simulink model "CARNOTews_M10C5_V1"  (Simulink 7.6)
settings: Solver=ode23tb  StartTime=t0  StopTime=t1
InitFcn:
  | tic;
  | parameter_CARNOTews;
StopFcn:
  | save(myfile,'simout');
  | save(myfile1,'simout1');
  | disp(['t_sim = ' num2str(toc/60) ' min'])
undefined symbols (not defined in the file or in its folder): Ad, Ad0, Ar, Au, Au0, Bd, Bd0, Bohrdurchmesser, Br, Bu, Bu0, c1, c33, c4, Cd, Cdl, Cr, Cu, Dd, DimAxi, DimRad, Dl, Dr, Du, fluid, gfunction, Gitterfaktor, Jahresmitteltemp, L1, lambdaErde, Massenstrom, mdot, mix, np, p0, Rechenradius, sample_time, Sondelaenge, Sondendurchmesser, T_null, t_start, Tdown_0, Tearth_anf, teta_in, TGrad, Ts_Trichter, Tup_0
libraries: carnot x2, simulink x1
settings Model: Creator=c8461075  LastModifiedBy=Fabian Ochs  SimulationMode=accelerator
settings OptimizationCC: InlineParams=on  SimCompilerOptimization=On
settings DebuggingCC: FcnCallInpInsideContextMsg=Enable All  UniqueDataStoreMsg=error

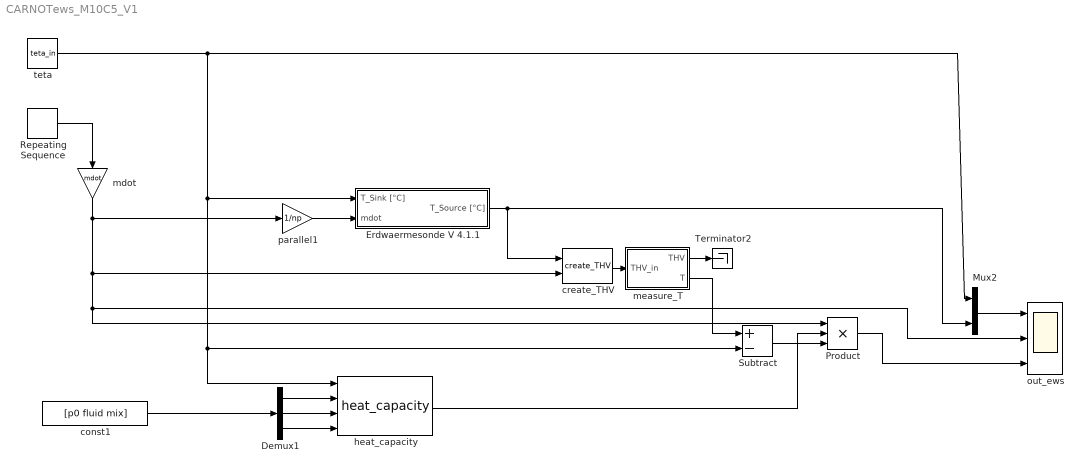
== system CARNOTews_M10C5_V1 ==
  Demux1 : Demux  Outputs=3
  Erdwaermesonde V 4.1.1 : Subsystem  mask{DimAxi=DimAxi, DimRad=DimRad, Jahresmitteltemp=Jahresmitteltemp, TGrad=TGrad, Massenstrom=Massenstrom, Sondendurchmesser=Sondendurchmesser, Bohrdurchmesser=Bohrdurchmesser, Sondelaenge=Sondelaenge, Rechenradius=Rechenradius, Gitterfaktor=Gitterfaktor}
      mask prompts: DimAxi "Knoten in axialer Richtung:"; DimRad "Knoten in radialer Richtung:"; Jahresmitteltemp "Jahresmitteltemperatur (K):"; TGrad "Temperaturgradient (K/m):"; Massenstrom "Massenstrom Sole (Kg/s):"; Sondendurchmesser "Sondendurchmesser (m):"; Bohrdurchmesser "Bohrdurchmesser (m):"; Sondelaenge "Sondenlänge (m):"; Rechenradius "Rechenradius (m):"
      mask help: Erdwärmesonde
      mask Help:
      | Anfangstemperatur T_PA: Verwendet die stationäre Temperaturverteilung der Erde und der Sole als Anfangstemperaturen im ganzen Gitter (Simulation fängt während der Heizsaison an).
      | Falls T_PA=-1 sind die Temperaturen der Erde in radialer Richtung konstant (die Simulation fängt am Anfang der Heizsaison an).
  Mux2 : Mux  Inputs=2
  Product : Product  Inputs=3  RndMeth=Zero
  Repeating Sequence : simulink/Sources/Repeating Sequence  SystemSampleTime=-1  rep_seq_t=[0 12 12 24]*3600  rep_seq_y=[1 1 0 0]
  Subtract : Sum  Inputs=+-
  Terminator2 : Terminator
  const1 : Constant  Value=[p0 fluid mix]
  create_THV : carnot/misc/create_THV  SystemSampleTime=-1  p=p0  fluid=water_glycol_mix  mix=mix  dia=0.02
  heat_capacity : carnot/materials/heat_capacity  SystemSampleTime=-1
  mdot : Gain  Gain=mdot
  measure_T : Subsystem  AncestorBlock=carnot/control/measure_T  mask(temperature measurement sensor){tc=10, t0=20}
      mask prompts: tc "time constant of sensor [s]"; t0 "initial temperature [degree centigrade]"
      mask help: Measurement sensor for temperatures with first-oder hold. Temperature is in degree centigrade.
      mask init:
      | tc = 1/max(tc, 0.001);
      mask Help: eval('man (''measure_T'')')
      mask Display: plot(-18,0,30,20,[0 20],[0 0],[10 10 8 8 12 12 10],[0 8 8 17 17 8 8],[10 10 9 9 11 11 10 9],[15 10 10 9 9 10 9 10])
  out_ews : Scope  NumInputPorts=3
      settings: TickLabels=on  YMin=1~0~0  YMax=11~0.5~37500  SaveName=simout  SampleInput=on  SampleTime=sample_time
  parallel1 : Gain  Gain=1/np
  teta : Constant  Value=teta_in
  wires:
  Mux2/1 -> out_ews/1
  Subtract/1 -> Product/3
  parallel1/1 -> Erdwaermesonde V 4.1.1/2(mdot)
  Erdwaermesonde V 4.1.1/1(T_Source [°C]) -> create_THV/1, Mux2/2
  create_THV/1 -> measure_T/1(THV_in)
  measure_T/2(T) -> Subtract/1
  measure_T/1(THV) -> Terminator2/1
  Demux1/1 -> heat_capacity/2
  Demux1/2 -> heat_capacity/3
  Demux1/3 -> heat_capacity/4
  teta/1 -> Erdwaermesonde V 4.1.1/1(T_Sink [°C]), heat_capacity/1, Subtract/2, Mux2/1
  const1/1 -> Demux1/1
  mdot/1 -> parallel1/1, create_THV/2, Product/1, out_ews/2
  heat_capacity/1 -> Product/2
  Product/1 -> out_ews/3
  Repeating Sequence/1 -> mdot/1

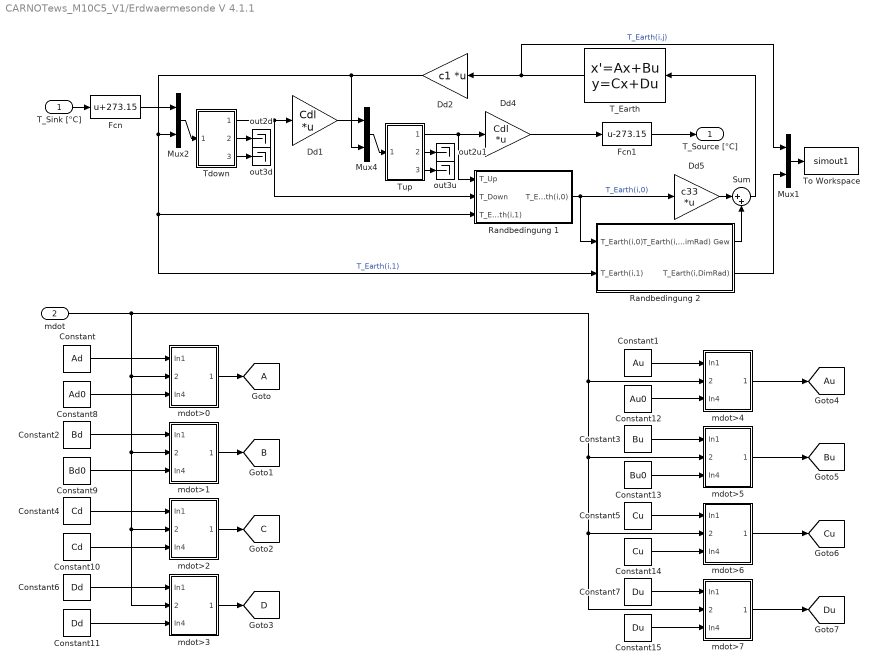
== system CARNOTews_M10C5_V1/Erdwaermesonde V 4.1.1 ==
  T_Sink [°C] : Inport
  mdot : Inport  Port=2
  Constant : Constant  Value=Ad
  Constant1 : Constant  Value=Au
  Constant10 : Constant  Value=Cd
  Constant11 : Constant  Value=Dd
  Constant12 : Constant  Value=Au0
  Constant13 : Constant  Value=Bu0
  Constant14 : Constant  Value=Cu
  Constant15 : Constant  Value=Du
  Constant2 : Constant  Value=Bd
  Constant3 : Constant  Value=Bu
  Constant4 : Constant  Value=Cd
  Constant5 : Constant  Value=Cu
  Constant6 : Constant  Value=Dd
  Constant7 : Constant  Value=Du
  Constant8 : Constant  Value=Ad0
  Constant9 : Constant  Value=Bd0
  Dd1 : Gain  Gain=Cdl  Multiplication=Matrix(K*u)  SaturateOnIntegerOverflow=on  OutDataTypeStr=Inherit: Same as input  ParamDataTypeStr=Inherit: Same as input
  Dd2 : Gain  Gain=c1  Multiplication=Matrix(K*u)  SaturateOnIntegerOverflow=on  OutDataTypeStr=Inherit: Same as input  ParamDataTypeStr=Inherit: Same as input
  Dd4 : Gain  Gain=Cdl  Multiplication=Matrix(K*u)  SaturateOnIntegerOverflow=on  OutDataTypeStr=Inherit: Same as input  ParamDataTypeStr=Inherit: Same as input
  Dd5 : Gain  Gain=c33  Multiplication=Matrix(K*u)  SaturateOnIntegerOverflow=on  OutDataTypeStr=Inherit: Same as input  ParamDataTypeStr=Inherit: Same as input
  Fcn : Fcn  Expr=u+273.15
  Fcn1 : Fcn  Expr=u-273.15
  Mux1 : Mux  Inputs=2
  Mux2 : Mux  Inputs=2
  Mux4 : Mux  Inputs=2
  Randbedingung 1 : Subsystem
  Randbedingung 2 : Subsystem
  Sum : Sum  Inputs=|++  SaturateOnIntegerOverflow=on  InputSameDT=on  OutDataTypeStr=Inherit: Same as first input
  T_Earth : StateSpace  A=Ar  B=Br  C=Cr  D=Dr  X0=Tearth_anf(:)
  Tdown : Subsystem
  To Workspace : ToWorkspace  VariableName=simout1  SampleTime=sample_time  SaveFormat=Structure With Time
  Tup : Subsystem
  mdot>0 : Subsystem
  mdot>1 : Subsystem
  mdot>2 : Subsystem
  mdot>3 : Subsystem
  mdot>4 : Subsystem
  mdot>5 : Subsystem
  mdot>6 : Subsystem
  mdot>7 : Subsystem
  out2d : Terminator
  out2u1 : Terminator
  out3d : Terminator
  out3u : Terminator
  T_Source [°C] : Outport
  tag scope: A=global, Au=global, B=global, Bu=global, C=global, Cu=global, D=global, Du=global
  wires:
  Fcn/1 -> Mux2/1
  Fcn1/1 -> T_Source [°C]/1
  Randbedingung 2/2(T_Earth(i,DimRad)) -> Mux1/2
  Dd2/1 -> Mux2/2, Randbedingung 1/3(T_Earth(i,1)), Randbedingung 2/2(T_Earth(i,1)), Mux4/2  "T_Earth(i,1)"
  Randbedingung 1/1(T_Earth(i,0)) -> Randbedingung 2/1(T_Earth(i,0)), Dd5/1  "T_Earth(i,0)"
  T_Sink [°C]/1 -> Fcn/1
  Sum/1 -> T_Earth/1
  Randbedingung 2/1(T_Earth(i,DimRad) Gew) -> Sum/2
  Dd5/1 -> Sum/1
  Dd4/1 -> Fcn1/1
  Tup/1(Out1) -> Dd4/1, Randbedingung 1/1(T_Up)
  T_Earth/1 -> Dd2/1, Mux1/1  "T_Earth(i,j)"
  Dd1/1 -> Mux4/1
  Mux4/1 -> Tup/1(In1)
  Mux2/1 -> Tdown/1(In1)
  Tdown/1(Out1) -> Dd1/1, Randbedingung 1/2(T_Down)
  Tdown/3(Out3) -> out3d/1
  Tup/3(Out3) -> out3u/1
  Tdown/2(Out2) -> out2d/1
  Tup/2(Out2) -> out2u1/1
  mdot>0/1(Out1) -> [A]
  Constant8/1 -> mdot>0/3(In4)
  mdot>1/1(Out1) -> [B]
  Constant/1 -> mdot>0/1(In1)
  Constant2/1 -> mdot>1/1(In1)
  Constant9/1 -> mdot>1/3(In4)
  mdot>2/1(Out1) -> [C]
  Constant4/1 -> mdot>2/1(In1)
  mdot>3/1(Out1) -> [D]
  Constant10/1 -> mdot>2/3(In4)
  Constant11/1 -> mdot>3/3(In4)
  Constant6/1 -> mdot>3/1(In1)
  Constant1/1 -> mdot>4/1(In1)
  Constant3/1 -> mdot>5/1(In1)
  Constant5/1 -> mdot>6/1(In1)
  Constant7/1 -> mdot>7/1(In1)
  mdot>7/1(Out1) -> [Du]
  mdot>6/1(Out1) -> [Cu]
  mdot>5/1(Out1) -> [Bu]
  mdot>4/1(Out1) -> [Au]
  Constant15/1 -> mdot>7/3(In4)
  Constant14/1 -> mdot>6/3(In4)
  Constant13/1 -> mdot>5/3(In4)
  Constant12/1 -> mdot>4/3(In4)
  mdot/1 -> mdot>0/2(mdot), mdot>1/2(mdot), mdot>2/2(mdot), mdot>3/2(mdot), mdot>4/2(mdot), mdot>5/2(mdot), mdot>6/2(mdot), mdot>7/2(mdot)
  Mux1/1 -> To Workspace/1

== system CARNOTews_M10C5_V1/measure_T ==
  THV_in : Inport
  heat capacity : StateSpace  A=-tc  B=tc  D=0  X0=t0
  select temperature : Selector  InputPortWidth=20  IndexOptions=Index vector (dialog)  Indices=[2]  OutputSizes=1
  THV : Outport  InitialOutput=0
  T : Outport  Port=2  InitialOutput=0
  wires:
  THV_in/1 -> select temperature/1, THV/1
  select temperature/1 -> heat capacity/1
  heat capacity/1 -> T/1

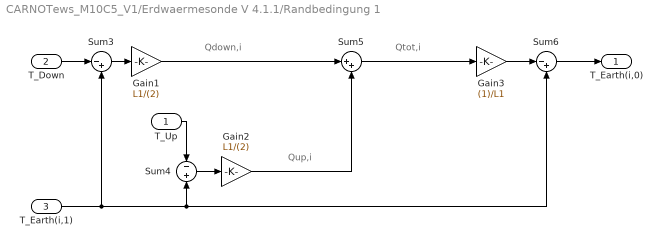
== system CARNOTews_M10C5_V1/Erdwaermesonde V 4.1.1/Randbedingung 1 ==
  note: Qtot,i
  note: Qup,i
  note: Qdown,i
  T_Up : Inport
  T_Down : Inport  Port=2
  T_Earth(i,1) : Inport  Port=3
  Gain1 : Gain  Gain=L1/(2)  SaturateOnIntegerOverflow=on  OutDataTypeStr=Inherit: Same as input  ParamDataTypeStr=Inherit: Same as input
  Gain2 : Gain  Gain=L1/(2)  SaturateOnIntegerOverflow=on  OutDataTypeStr=Inherit: Same as input  ParamDataTypeStr=Inherit: Same as input
  Gain3 : Gain  Gain=(1)/L1  SaturateOnIntegerOverflow=on  OutDataTypeStr=Inherit: Same as input  ParamDataTypeStr=Inherit: Same as input
  Sum3 : Sum  Inputs=|-+  SaturateOnIntegerOverflow=on  InputSameDT=on  OutDataTypeStr=Inherit: Same as first input
  Sum4 : Sum  Inputs=-+  SaturateOnIntegerOverflow=on  InputSameDT=on  OutDataTypeStr=Inherit: Same as first input
  Sum5 : Sum  Inputs=|++  SaturateOnIntegerOverflow=on  InputSameDT=on  OutDataTypeStr=Inherit: Same as first input
  Sum6 : Sum  Inputs=|-+  SaturateOnIntegerOverflow=on  InputSameDT=on  OutDataTypeStr=Inherit: Same as first input
  T_Earth(i,0) : Outport
  wires:
  Sum6/1 -> T_Earth(i,0)/1
  T_Earth(i,1)/1 -> Sum6/2, Sum4/2, Sum3/2
  T_Up/1 -> Sum4/1
  T_Down/1 -> Sum3/1
  Gain3/1 -> Sum6/1
  Sum5/1 -> Gain3/1
  Gain2/1 -> Sum5/2
  Gain1/1 -> Sum5/1
  Sum4/1 -> Gain2/1
  Sum3/1 -> Gain1/1

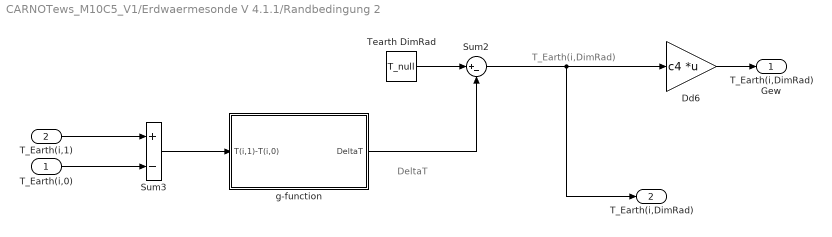
== system CARNOTews_M10C5_V1/Erdwaermesonde V 4.1.1/Randbedingung 2 ==
  note: DeltaT
  note: T_Earth(i,DimRad)
  T_Earth(i,0) : Inport
  T_Earth(i,1) : Inport  Port=2
  Dd6 : Gain  Gain=c4  Multiplication=Matrix(K*u)  SaturateOnIntegerOverflow=on  OutDataTypeStr=Inherit: Same as input  ParamDataTypeStr=Inherit: Same as input
  Sum2 : Sum  Inputs=|+-  SaturateOnIntegerOverflow=on  InputSameDT=on  OutDataTypeStr=Inherit: Same as first input
  Sum3 : Sum  Inputs=+-  SaturateOnIntegerOverflow=on  InputSameDT=on  OutDataTypeStr=Inherit: Same as first input
  Tearth DimRad : Constant  Value=T_null  VectorParams1D=off
  g-function : Subsystem
  T_Earth(i,DimRad) Gew : Outport
  T_Earth(i,DimRad) : Outport  Port=2
  wires:
  g-function/1(DeltaT) -> Sum2/2
  Sum3/1 -> g-function/1(T(i,1)-T(i,0))
  Dd6/1 -> T_Earth(i,DimRad) Gew/1
  T_Earth(i,0)/1 -> Sum3/2
  T_Earth(i,1)/1 -> Sum3/1
  Tearth DimRad/1 -> Sum2/1
  Sum2/1 -> T_Earth(i,DimRad)/1, Dd6/1

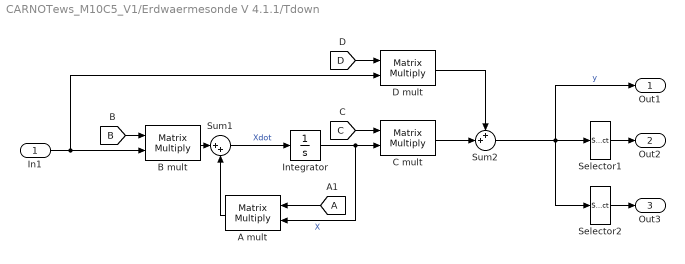
== system CARNOTews_M10C5_V1/Erdwaermesonde V 4.1.1/Tdown ==
  In1 : Inport
  A mult : Product  Multiplication=Matrix(*)  RndMeth=Zero
  B mult : Product  Multiplication=Matrix(*)  RndMeth=Zero
  C mult : Product  Multiplication=Matrix(*)  RndMeth=Zero
  D mult : Product  Multiplication=Matrix(*)  RndMeth=Zero
  Integrator : Integrator  InitialCondition=Tdown_0
  Selector1 : Selector  InputPortWidth=DimAxi/2  IndexOptions=Index vector (dialog)  Indices=1  OutputSizes=1
  Selector2 : Selector  InputPortWidth=DimAxi/2  IndexOptions=Index vector (dialog)  Indices=2  OutputSizes=1
  Sum1 : Sum  Inputs=|++
  Sum2 : Sum  Inputs=++|
  Out1 : Outport
  Out2 : Outport  Port=2
  Out3 : Outport  Port=3
  wires:
  Sum2/1 -> Selector2/1, Selector1/1, Out1/1  "y"
  In1/1 -> B mult/2, D mult/2
  D mult/1 -> Sum2/1
  C mult/1 -> Sum2/2
  B mult/1 -> Sum1/1
  Sum1/1 -> Integrator/1  "Xdot"
  Integrator/1 -> A mult/2, C mult/2  "X"
  A mult/1 -> Sum1/2
  [B] -> B mult/1
  [A] -> A mult/1
  [C] -> C mult/1
  [D] -> D mult/1
  Selector1/1 -> Out2/1
  Selector2/1 -> Out3/1

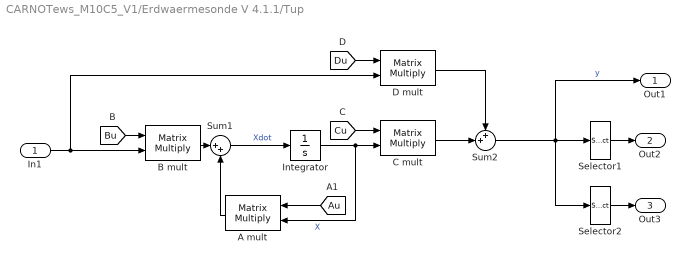
== system CARNOTews_M10C5_V1/Erdwaermesonde V 4.1.1/Tup ==
  In1 : Inport
  A mult : Product  Multiplication=Matrix(*)  RndMeth=Zero
  B mult : Product  Multiplication=Matrix(*)  RndMeth=Zero
  C mult : Product  Multiplication=Matrix(*)  RndMeth=Zero
  D mult : Product  Multiplication=Matrix(*)  RndMeth=Zero
  Integrator : Integrator  InitialCondition=Tup_0
  Selector1 : Selector  InputPortWidth=DimAxi/2  IndexOptions=Index vector (dialog)  Indices=1  OutputSizes=1
  Selector2 : Selector  InputPortWidth=DimAxi/2  IndexOptions=Index vector (dialog)  Indices=2  OutputSizes=1
  Sum1 : Sum  Inputs=|++
  Sum2 : Sum  Inputs=++|
  Out1 : Outport
  Out2 : Outport  Port=2
  Out3 : Outport  Port=3
  wires:
  Sum2/1 -> Selector2/1, Selector1/1, Out1/1  "y"
  In1/1 -> B mult/2, D mult/2
  D mult/1 -> Sum2/1
  C mult/1 -> Sum2/2
  B mult/1 -> Sum1/1
  Sum1/1 -> Integrator/1  "Xdot"
  Integrator/1 -> A mult/2, C mult/2  "X"
  A mult/1 -> Sum1/2
  [Bu] -> B mult/1
  [Au] -> A mult/1
  [Cu] -> C mult/1
  [Du] -> D mult/1
  Selector1/1 -> Out2/1
  Selector2/1 -> Out3/1

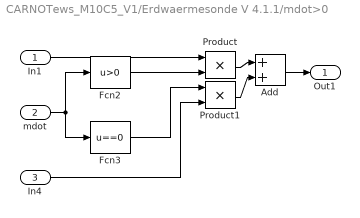
== system CARNOTews_M10C5_V1/Erdwaermesonde V 4.1.1/mdot>0 ==
  In1 : Inport
  mdot : Inport  Port=2
  In4 : Inport  Port=3
  Add : Sum
  Fcn2 : Fcn  Expr=u>0
  Fcn3 : Fcn  Expr=u==0
  Product : Product  RndMeth=Zero
  Product1 : Product  RndMeth=Zero
  Out1 : Outport
  wires:
  Product/1 -> Add/1
  Product1/1 -> Add/2
  In1/1 -> Product/1
  Add/1 -> Out1/1
  In4/1 -> Product1/2
  mdot/1 -> Fcn2/1, Fcn3/1
  Fcn2/1 -> Product/2
  Fcn3/1 -> Product1/1

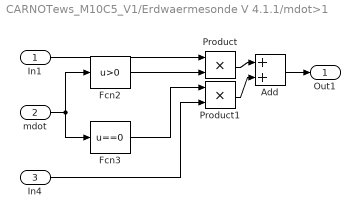
== system CARNOTews_M10C5_V1/Erdwaermesonde V 4.1.1/mdot>1 ==
  In1 : Inport
  mdot : Inport  Port=2
  In4 : Inport  Port=3
  Add : Sum
  Fcn2 : Fcn  Expr=u>0
  Fcn3 : Fcn  Expr=u==0
  Product : Product  RndMeth=Zero
  Product1 : Product  RndMeth=Zero
  Out1 : Outport
  wires:
  Product/1 -> Add/1
  Product1/1 -> Add/2
  In1/1 -> Product/1
  Add/1 -> Out1/1
  In4/1 -> Product1/2
  mdot/1 -> Fcn2/1, Fcn3/1
  Fcn2/1 -> Product/2
  Fcn3/1 -> Product1/1

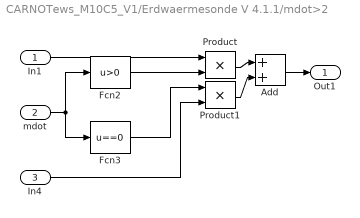
== system CARNOTews_M10C5_V1/Erdwaermesonde V 4.1.1/mdot>2 ==
  In1 : Inport
  mdot : Inport  Port=2
  In4 : Inport  Port=3
  Add : Sum
  Fcn2 : Fcn  Expr=u>0
  Fcn3 : Fcn  Expr=u==0
  Product : Product  RndMeth=Zero
  Product1 : Product  RndMeth=Zero
  Out1 : Outport
  wires:
  Product/1 -> Add/1
  Product1/1 -> Add/2
  In1/1 -> Product/1
  Add/1 -> Out1/1
  In4/1 -> Product1/2
  mdot/1 -> Fcn2/1, Fcn3/1
  Fcn2/1 -> Product/2
  Fcn3/1 -> Product1/1

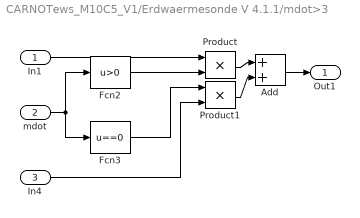
== system CARNOTews_M10C5_V1/Erdwaermesonde V 4.1.1/mdot>3 ==
  In1 : Inport
  mdot : Inport  Port=2
  In4 : Inport  Port=3
  Add : Sum
  Fcn2 : Fcn  Expr=u>0
  Fcn3 : Fcn  Expr=u==0
  Product : Product  RndMeth=Zero
  Product1 : Product  RndMeth=Zero
  Out1 : Outport
  wires:
  Product/1 -> Add/1
  Product1/1 -> Add/2
  In1/1 -> Product/1
  Add/1 -> Out1/1
  In4/1 -> Product1/2
  mdot/1 -> Fcn2/1, Fcn3/1
  Fcn2/1 -> Product/2
  Fcn3/1 -> Product1/1

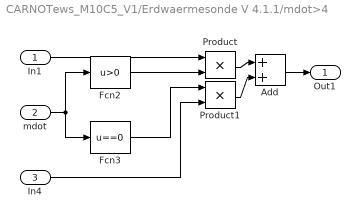
== system CARNOTews_M10C5_V1/Erdwaermesonde V 4.1.1/mdot>4 ==
  In1 : Inport
  mdot : Inport  Port=2
  In4 : Inport  Port=3
  Add : Sum
  Fcn2 : Fcn  Expr=u>0
  Fcn3 : Fcn  Expr=u==0
  Product : Product  RndMeth=Zero
  Product1 : Product  RndMeth=Zero
  Out1 : Outport
  wires:
  Product/1 -> Add/1
  Product1/1 -> Add/2
  In1/1 -> Product/1
  Add/1 -> Out1/1
  In4/1 -> Product1/2
  mdot/1 -> Fcn2/1, Fcn3/1
  Fcn2/1 -> Product/2
  Fcn3/1 -> Product1/1

== system CARNOTews_M10C5_V1/Erdwaermesonde V 4.1.1/mdot>5 ==
  In1 : Inport
  mdot : Inport  Port=2
  In4 : Inport  Port=3
  Add : Sum
  Fcn2 : Fcn  Expr=u>0
  Fcn3 : Fcn  Expr=u==0
  Product : Product  RndMeth=Zero
  Product1 : Product  RndMeth=Zero
  Out1 : Outport
  wires:
  Product/1 -> Add/1
  Product1/1 -> Add/2
  In1/1 -> Product/1
  Add/1 -> Out1/1
  In4/1 -> Product1/2
  mdot/1 -> Fcn2/1, Fcn3/1
  Fcn2/1 -> Product/2
  Fcn3/1 -> Product1/1

== system CARNOTews_M10C5_V1/Erdwaermesonde V 4.1.1/mdot>6 ==
  In1 : Inport
  mdot : Inport  Port=2
  In4 : Inport  Port=3
  Add : Sum
  Fcn2 : Fcn  Expr=u>0
  Fcn3 : Fcn  Expr=u==0
  Product : Product  RndMeth=Zero
  Product1 : Product  RndMeth=Zero
  Out1 : Outport
  wires:
  Product/1 -> Add/1
  Product1/1 -> Add/2
  In1/1 -> Product/1
  Add/1 -> Out1/1
  In4/1 -> Product1/2
  mdot/1 -> Fcn2/1, Fcn3/1
  Fcn2/1 -> Product/2
  Fcn3/1 -> Product1/1

== system CARNOTews_M10C5_V1/Erdwaermesonde V 4.1.1/mdot>7 ==
  In1 : Inport
  mdot : Inport  Port=2
  In4 : Inport  Port=3
  Add : Sum
  Fcn2 : Fcn  Expr=u>0
  Fcn3 : Fcn  Expr=u==0
  Product : Product  RndMeth=Zero
  Product1 : Product  RndMeth=Zero
  Out1 : Outport
  wires:
  Product/1 -> Add/1
  Product1/1 -> Add/2
  In1/1 -> Product/1
  Add/1 -> Out1/1
  In4/1 -> Product1/2
  mdot/1 -> Fcn2/1, Fcn3/1
  Fcn2/1 -> Product/2
  Fcn3/1 -> Product1/1

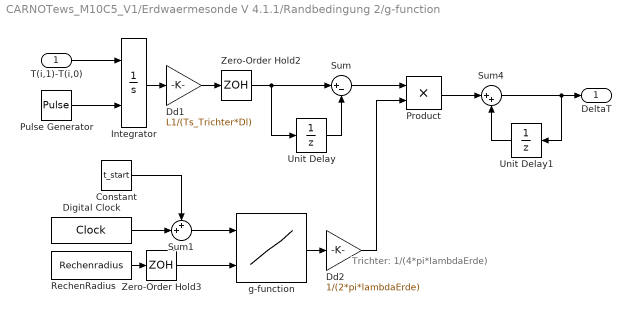
== system CARNOTews_M10C5_V1/Erdwaermesonde V 4.1.1/Randbedingung 2/g-function ==
  note: Trichter: 1/(4*pi*lambdaErde)
  T(i,1)-T(i,0) : Inport
  Constant : Constant  Value=t_start
  Dd1 : Gain  Gain=L1/(Ts_Trichter*Dl)  SaturateOnIntegerOverflow=on  OutDataTypeStr=Inherit: Same as input  ParamDataTypeStr=Inherit: Same as input
  Dd2 : Gain  Gain=1/(2*pi*lambdaErde)  SaturateOnIntegerOverflow=on  OutDataTypeStr=Inherit: Same as input  ParamDataTypeStr=Inherit: Same as input
  Digital Clock : DigitalClock
  Integrator : Integrator  ExternalReset=rising
  Product : Product  SaturateOnIntegerOverflow=on  RndMeth=Zero  InputSameDT=on  OutDataTypeStr=Inherit: Same as first input
  Pulse Generator : DiscretePulseGenerator  PulseType=Time based  Period=Ts_Trichter  PulseWidth=50  PhaseDelay=300
  RechenRadius : Constant  Value=Rechenradius  VectorParams1D=off
  Sum : Sum  Inputs=|+-  SaturateOnIntegerOverflow=on  InputSameDT=on  OutDataTypeStr=Inherit: Same as first input
  Sum1 : Sum  Inputs=++|  SaturateOnIntegerOverflow=on  InputSameDT=on  OutDataTypeStr=Inherit: Same as first input
  Sum4 : Sum  Inputs=|++  SaturateOnIntegerOverflow=on  InputSameDT=on  OutDataTypeStr=Inherit: Same as first input
  Unit Delay : UnitDelay
  Unit Delay1 : UnitDelay
  Zero-Order Hold2 : ZeroOrderHold
  Zero-Order Hold3 : ZeroOrderHold
  g-function : Lookup2D  RowIndex=t_Trichter  ColumnIndex=r_Trichter  Table=gfunction  SaturateOnIntegerOverflow=on  InputSameDT=on
  DeltaT : Outport
  wires:
  T(i,1)-T(i,0)/1 -> Integrator/1
  Zero-Order Hold2/1 -> Sum/1, Unit Delay/1
  Zero-Order Hold3/1 -> g-function/2
  Sum4/1 -> DeltaT/1, Unit Delay1/1
  Unit Delay1/1 -> Sum4/2
  Dd2/1 -> Product/2
  Product/1 -> Sum4/1
  RechenRadius/1 -> Zero-Order Hold3/1
  g-function/1 -> Dd2/1
  Sum/1 -> Product/1
  Unit Delay/1 -> Sum/2
  Dd1/1 -> Zero-Order Hold2/1
  Integrator/1 -> Dd1/1
  Pulse Generator/1 -> Integrator/2
  Digital Clock/1 -> Sum1/2
  Sum1/1 -> g-function/1
  Constant/1 -> Sum1/1
